simulink model "QuarterCarModel2"  (R2024a)
settings: Solver=VariableStepAuto  StartTime=0.0  StopTime=10.0  RelTol=1e-3
settings Model: Creator=LENOVO  LastModifiedBy=LENOVO

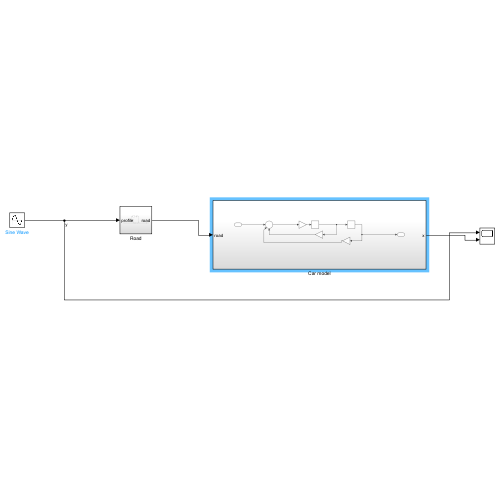
[thumbnail: Simulink's stored preview of the top-level diagram]
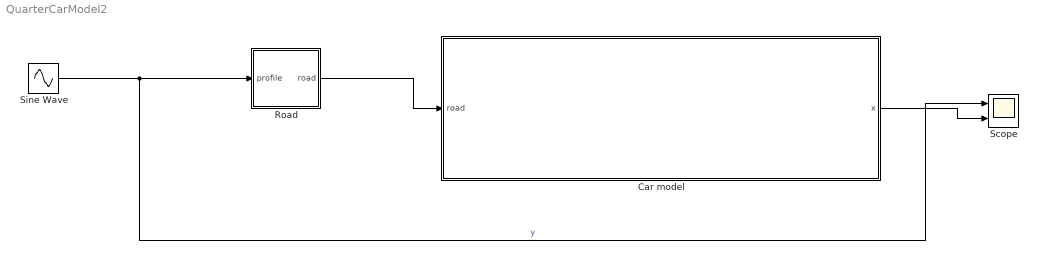
== system QuarterCarModel2 ==
  Car model : Subsystem
  Road : Subsystem
  Scope : Scope  NumInputPorts=2
  Sine Wave : Sin  Amplitude=0.1  Frequency=0.5  SampleTime=0
  wires:
  Sine Wave/1 -> Road/1(profile), Scope/1  "y"
  Road/1(road) -> Car model/1(road)
  Car model/1(x) -> Scope/2

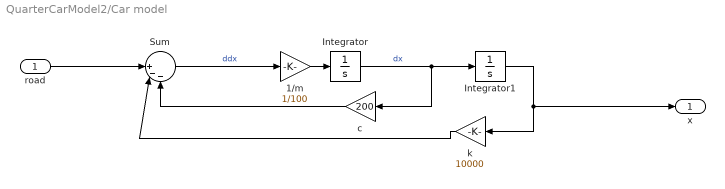
== system QuarterCarModel2/Car model ==
  road : Inport
  1/m : Gain  Gain=1/100
  Integrator : Integrator
  Integrator1 : Integrator
  Sum : Sum  Inputs=||+--
  c : Gain  Gain=200
  k : Gain  Gain=10000
  x : Outport
  wires:
  Sum/1 -> 1/m/1  "ddx"
  Integrator/1 -> c/1, Integrator1/1  "dx"
  1/m/1 -> Integrator/1
  k/1 -> Sum/2
  Integrator1/1 -> x/1, k/1
  c/1 -> Sum/3
  road/1 -> Sum/1

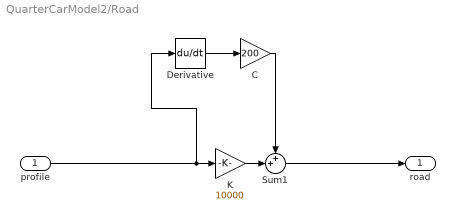
== system QuarterCarModel2/Road ==
  profile : Inport
  C : Gain  Gain=200
  Derivative : Derivative
  K : Gain  Gain=10000
  Sum1 : Sum  Inputs=++|
  road : Outport
  wires:
  profile/1 -> Derivative/1, K/1
  C/1 -> Sum1/1
  Derivative/1 -> C/1
  K/1 -> Sum1/2
  Sum1/1 -> road/1
